simulink library "hcu_lib"  (Simulink 8.6)
settings: Solver=ode45  SolverMode=SingleTasking  StartTime=0.0  StopTime=10.0  RelTol=1e-3
PreLoadFcn:
  | if exist('tl_preloadfcn','file'), tl_preloadfcn(gcs,100); end
PostLoadFcn:
  | if exist('tl_postloadfcn','file'), tl_postloadfcn(gcs,100); end
undefined symbols (not defined in the file or in its folder): C_TICK_TIME_S, DEG2RAD, EPSILON, FALSE, RAD2DEG, TRUE
undefined symbols (not defined in the file): UNDEFINED_VALUE
libraries: hcu_lib x19, simulink x4
(part 2 of 3)

== system hcu_lib/P_Controller ==
  note: P Controller
  TargetValue : Inport
  FeedbackValue : Inport  Port=2
  FeedForward : Inport  Port=3
  Error_Gain : Inport  Port=4
  P_Gain : Inport  Port=5
  ControlHold : Inport  Port=6
  Constant14 : Constant  Value=single(0)
  Data Type Conversion : DataTypeConversion  OutDataTypeStr=single  SaturateOnIntegerOverflow=on  RndMeth=Zero
  Product2 : Product  InputSameDT=on  OutDataTypeStr=Inherit: Same as first input
  Product3 : Product  InputSameDT=on  OutDataTypeStr=Inherit: Same as first input
  Sum1 : Sum  Inputs=++|
  Sum2 : Sum  Inputs=+|-  SaturateOnIntegerOverflow=on  InputSameDT=on  OutDataTypeStr=Inherit: Same as first input
  Switch2 : Switch  Criteria=u2 ~= 0
  Switch4 : Switch  Criteria=u2 ~= 0
  Unit Delay1 : UnitDelay  SampleTime=-1
  Out : Outport  OutputWhenDisabled=reset  InitialOutput=[0]
  Control_Error : Outport  Port=2  OutputWhenDisabled=reset  InitialOutput=[0]
  P_term : Outport  Port=3  OutputWhenDisabled=reset  InitialOutput=[0]
  wires:
  FeedbackValue/1 -> Sum2/2
  TargetValue/1 -> Sum2/1
  Error_Gain/1 -> Product3/2
  P_Gain/1 -> Product2/1
  Product2/1 -> Sum1/2, P_term/1
  Product3/1 -> Product2/2
  Sum2/1 -> Data Type Conversion/1
  ControlHold/1 -> [HoldReq]
  [HoldReq] -> Switch2/2
  Switch2/1 -> Out/1, Unit Delay1/1
  Unit Delay1/1 -> Switch2/1
  Switch4/1 -> Product3/1
  Data Type Conversion/1 -> Control_Error/1, Switch4/3
  [HoldReq] -> Switch4/2
  Constant14/1 -> Switch4/1
  Sum1/1 -> Switch2/3
  FeedForward/1 -> Sum1/1

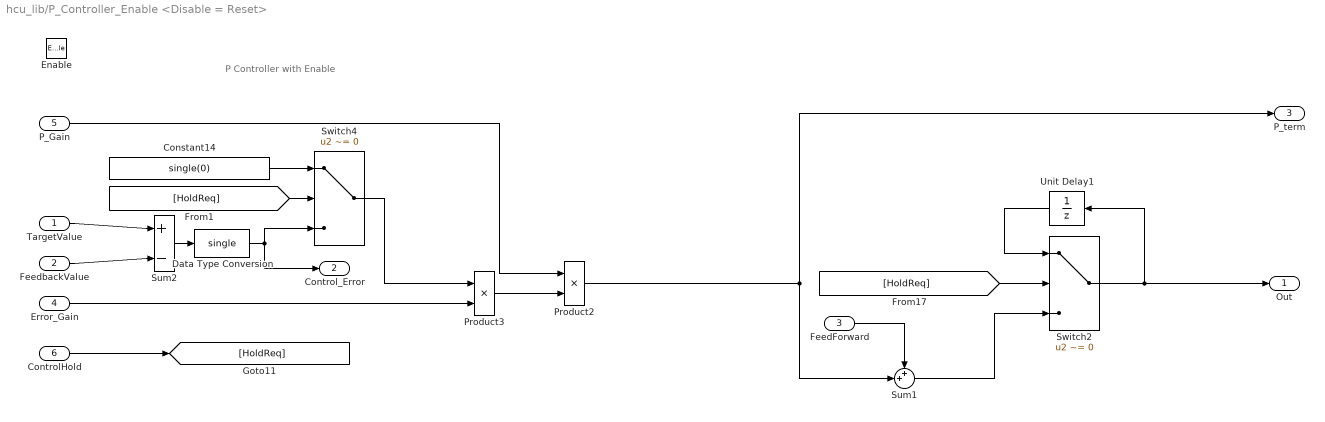
== system hcu_lib/P_Controller_Enable <Disable = Reset> ==
  note: P Controller with Enable
  TargetValue : Inport
  FeedbackValue : Inport  Port=2
  FeedForward : Inport  Port=3
  Error_Gain : Inport  Port=4
  P_Gain : Inport  Port=5
  ControlHold : Inport  Port=6
  Enable : EnablePort  StatesWhenEnabling=reset
  Constant14 : Constant  Value=single(0)
  Data Type Conversion : DataTypeConversion  OutDataTypeStr=single  SaturateOnIntegerOverflow=on  RndMeth=Zero
  Product2 : Product  InputSameDT=on  OutDataTypeStr=Inherit: Same as first input
  Product3 : Product  InputSameDT=on  OutDataTypeStr=Inherit: Same as first input
  Sum1 : Sum  Inputs=++|
  Sum2 : Sum  Inputs=+|-  SaturateOnIntegerOverflow=on  InputSameDT=on  OutDataTypeStr=Inherit: Same as first input
  Switch2 : Switch  Criteria=u2 ~= 0
  Switch4 : Switch  Criteria=u2 ~= 0
  Unit Delay1 : UnitDelay  SampleTime=-1
  Out : Outport  OutputWhenDisabled=reset  InitialOutput=[0]
  Control_Error : Outport  Port=2  OutputWhenDisabled=reset  InitialOutput=[0]
  P_term : Outport  Port=3  OutputWhenDisabled=reset  InitialOutput=[0]
  wires:
  FeedForward/1 -> Sum1/1
  Sum1/1 -> Switch2/3
  Constant14/1 -> Switch4/1
  [HoldReq] -> Switch4/2
  Data Type Conversion/1 -> Switch4/3, Control_Error/1
  Switch4/1 -> Product3/1
  Unit Delay1/1 -> Switch2/1
  Switch2/1 -> Unit Delay1/1, Out/1
  [HoldReq] -> Switch2/2
  ControlHold/1 -> [HoldReq]
  Sum2/1 -> Data Type Conversion/1
  Product3/1 -> Product2/2
  Product2/1 -> P_term/1, Sum1/2
  P_Gain/1 -> Product2/1
  Error_Gain/1 -> Product3/2
  TargetValue/1 -> Sum2/1
  FeedbackValue/1 -> Sum2/2

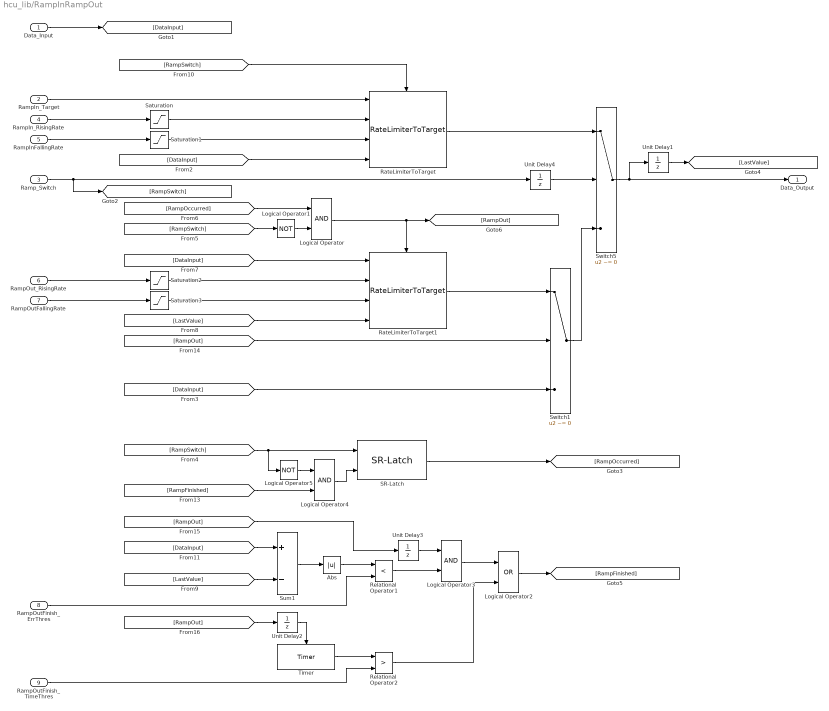
== system hcu_lib/RampInRampOut ==
  Data_Input : Inport
  RampIn_Target : Inport  Port=2
  Ramp_Switch : Inport  Port=3
  RampIn_RisingRate : Inport  Port=4
  RampInFallingRate : Inport  Port=5
  RampOut_RisingRate : Inport  Port=6
  RampOutFallingRate : Inport  Port=7
  RampOutFinish_ErrThres : Inport  Port=8
  RampOutFinish_TimeThres : Inport  Port=9
  Abs : Abs
  Logical Operator : Logic  AllPortsSameDT=off  OutDataTypeStr=boolean
  Logical Operator1 : Logic  Operator=NOT  AllPortsSameDT=off  OutDataTypeStr=boolean
  Logical Operator2 : Logic  Operator=OR  AllPortsSameDT=off  OutDataTypeStr=boolean
  Logical Operator3 : Logic  AllPortsSameDT=off  OutDataTypeStr=boolean
  Logical Operator4 : Logic  AllPortsSameDT=off  OutDataTypeStr=boolean
  Logical Operator5 : Logic  Operator=NOT  AllPortsSameDT=off  OutDataTypeStr=boolean
  RateLimiterToTarget : hcu_lib/RateLimiterToTarget  SystemSampleTime=-1
  RateLimiterToTarget1 : hcu_lib/RateLimiterToTarget  SystemSampleTime=-1
  Relational Operator1 : RelationalOperator  Operator=<  OutDataTypeStr=boolean
  Relational Operator2 : RelationalOperator  Operator=>  OutDataTypeStr=boolean
  SR-Latch : hcu_lib/SR-Latch  SystemSampleTime=-1
  Saturation : Saturate  UpperLimit=inf  LowerLimit=0
  Saturation1 : Saturate  UpperLimit=0  LowerLimit=-inf
  Saturation2 : Saturate  UpperLimit=inf  LowerLimit=0
  Saturation3 : Saturate  UpperLimit=0  LowerLimit=-inf
  Sum1 : Sum  Inputs=+-
  Switch1 : Switch  Criteria=u2 ~= 0
  Switch5 : Switch  Criteria=u2 ~= 0
  Timer : hcu_lib/Timer  SystemSampleTime=-1
  Unit Delay{1..4} (4 alike) : UnitDelay  SampleTime=-1
  Data_Output : Outport  InitialOutput=[0]
  wires:
  Data_Input/1 -> [DataInput]
  RateLimiterToTarget/1 -> Switch5/1
  [RampSwitch] -> RateLimiterToTarget/Enable
  RampIn_Target/1 -> RateLimiterToTarget/1
  RampIn_RisingRate/1 -> Saturation/1
  RampInFallingRate/1 -> Saturation1/1
  [DataInput] -> RateLimiterToTarget/4
  [DataInput] -> Switch1/3
  Switch5/1 -> Unit Delay1/1, Data_Output/1
  [RampSwitch] -> SR-Latch/1, Logical Operator5/1
  SR-Latch/1 -> [RampOccurred]
  Switch1/1 -> Switch5/3
  [RampSwitch] -> Logical Operator1/1
  [RampOccurred] -> Logical Operator/1
  Logical Operator1/1 -> Logical Operator/2
  [DataInput] -> RateLimiterToTarget1/1
  RampOut_RisingRate/1 -> Saturation2/1
  RampOutFallingRate/1 -> Saturation3/1
  [LastValue] -> RateLimiterToTarget1/4
  Unit Delay1/1 -> [LastValue]
  [DataInput] -> Sum1/1
  [LastValue] -> Sum1/2
  Sum1/1 -> Abs/1
  Abs/1 -> Relational Operator1/1
  RampOutFinish_ErrThres/1 -> Relational Operator1/2
  [RampOut] -> Unit Delay2/1
  Timer/1 -> Relational Operator2/1
  RampOutFinish_TimeThres/1 -> Relational Operator2/2
  Relational Operator1/1 -> Logical Operator3/2
  Relational Operator2/1 -> Logical Operator2/2
  Logical Operator2/1 -> [RampFinished]
  [RampFinished] -> Logical Operator4/2
  Unit Delay2/1 -> Timer/Enable
  Logical Operator3/1 -> Logical Operator2/1
  Logical Operator5/1 -> Logical Operator4/1
  Logical Operator4/1 -> SR-Latch/2
  Logical Operator/1 -> RateLimiterToTarget1/Enable, [RampOut]
  Ramp_Switch/1 -> Unit Delay4/1, [RampSwitch]
  RateLimiterToTarget1/1 -> Switch1/1
  Unit Delay4/1 -> Switch5/2
  [RampOut] -> Switch1/2
  Unit Delay3/1 -> Logical Operator3/1
  [RampOut] -> Unit Delay3/1
  Saturation/1 -> RateLimiterToTarget/2
  Saturation1/1 -> RateLimiterToTarget/3
  Saturation3/1 -> RateLimiterToTarget1/3
  Saturation2/1 -> RateLimiterToTarget1/2

== system hcu_lib/RateLimit ==
  input_raw : Inport
  steptime : Inport  Port=2
  ratelimt_inc : Inport  Port=3
  ratelimt_dec : Inport  Port=4
  MinMax : MinMax  Inputs=2
  MinMax1 : MinMax  Function=max  Inputs=2
  MinMax2 : MinMax  Function=max  Inputs=2
  MinMax3 : MinMax  Inputs=2
  Product : Product  RndMeth=Zero
  Product1 : Product  RndMeth=Zero
  Sum5 : Sum  Inputs=+-
  Sum6 : Sum
  UnitDelay1 : UnitDelay  SampleTime=-1
  step_time6 : Constant  Value=0  OutDataTypeStr=single
  output : Outport
  wires:
  ratelimt_dec/1 -> Product1/2
  steptime/1 -> Product1/1, Product/2
  Sum5/1 -> MinMax1/1
  [Dec] -> MinMax1/2
  [Inc] -> MinMax/1
  MinMax1/1 -> MinMax/2
  MinMax/1 -> Sum6/1
  input_raw/1 -> Sum5/1
  Sum6/1 -> output/1, UnitDelay1/1
  UnitDelay1/1 -> Sum5/2, Sum6/2
  Product/1 -> MinMax2/1
  Product1/1 -> MinMax3/2
  step_time6/1 -> MinMax2/2, MinMax3/1
  MinMax2/1 -> [Inc]
  MinMax3/1 -> [Dec]
  ratelimt_inc/1 -> Product/1

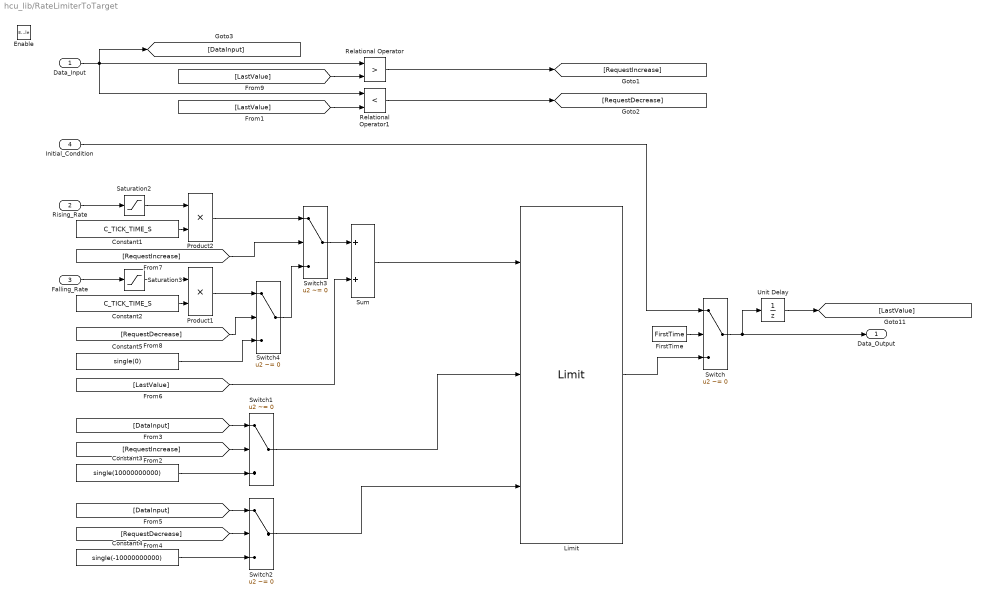
== system hcu_lib/RateLimiterToTarget ==
  Data_Input : Inport
  Rising_Rate : Inport  Port=2
  Falling_Rate : Inport  Port=3
  Initial_Condition : Inport  Port=4
  Enable : EnablePort  StatesWhenEnabling=reset
  Constant1 : Constant  Value=C_TICK_TIME_S
  Constant2 : Constant  Value=C_TICK_TIME_S
  Constant3 : Constant  Value=single(10000000000)
  Constant4 : Constant  Value=single(-10000000000)
  Constant5 : Constant  Value=single(0)
  FirstTime : hcu_lib/FirstTime
  Limit : hcu_lib/Limit  SystemSampleTime=-1
  Product1 : Product  Inputs=**  RndMeth=Zero
  Product2 : Product  Inputs=**  RndMeth=Zero
  Relational Operator : RelationalOperator  Operator=>  OutDataTypeStr=boolean
  Relational Operator1 : RelationalOperator  Operator=<  OutDataTypeStr=boolean
  Saturation2 : Saturate  UpperLimit=inf  LowerLimit=0
  Saturation3 : Saturate  UpperLimit=0  LowerLimit=-inf
  Sum : Sum
  Switch{,1..4} (5 alike) : Switch  Criteria=u2 ~= 0
  Unit Delay : UnitDelay  SampleTime=-1
  Data_Output : Outport  InitialOutput=[0]
  wires:
  Limit/1 -> Switch/3
  Saturation3/1 -> Product1/1
  Saturation2/1 -> Product2/1
  Constant5/1 -> Switch4/3
  Product1/1 -> Switch4/1
  Switch4/1 -> Switch3/3
  [RequestDecrease] -> Switch4/2
  Switch3/1 -> Sum/1
  Product2/1 -> Switch3/1
  [LastValue] -> Sum/2
  [RequestIncrease] -> Switch3/2
  Switch2/1 -> Limit/3
  Switch1/1 -> Limit/2
  [DataInput] -> Switch2/1
  Constant4/1 -> Switch2/3
  [RequestDecrease] -> Switch2/2
  Constant3/1 -> Switch1/3
  [DataInput] -> Switch1/1
  [RequestIncrease] -> Switch1/2
  Switch/1 -> Data_Output/1, Unit Delay/1
  Relational Operator1/1 -> [RequestDecrease]
  [LastValue] -> Relational Operator1/2
  Data_Input/1 -> Relational Operator1/1, Relational Operator/1, [DataInput]
  Relational Operator/1 -> [RequestIncrease]
  [LastValue] -> Relational Operator/2
  Unit Delay/1 -> [LastValue]
  Falling_Rate/1 -> Saturation3/1
  Constant2/1 -> Product1/2
  Rising_Rate/1 -> Saturation2/1
  Sum/1 -> Limit/1
  Initial_Condition/1 -> Switch/1
  FirstTime/1 -> Switch/2
  Constant1/1 -> Product2/2

== system hcu_lib/ReqId ==

== system hcu_lib/SIN ==
  u_rad : Inport
  Constant : Constant  Value=single(2*pi)
  Gain : Gain  Gain=2*pi
  Product : Product  Inputs=*/
  Rounding Function : Rounding
  SIN_Function : Lookup_n-D  NumberOfTableDimensions=1  BreakpointsForDimension1="[0\t5\t10\t15\t30\t45\t60\t75\t80\t85\t90\t95\t100\t105\t120\t135\t150\t165\t170\t175\t180\t185\t190\t195\t210\t225\t240\t255\t260\t265\t270\t275\t280\t285\t300\t315\t330\t345\t350\t355\t360]"  Table="[0\t0.087155743\t0.173648178\t0.258819045\t0.5\t0.707106781\t0.866025404\t0.965925826\t0.984807753\t0.996194698\t1\t0.996194698\t0.984807753\t0.965925826\t0.866025404\t0.707106781\t0.5\t0.258819045\t0.173648178\t0.087155743\t0\t-0.087155743\t-0.173648178\t-0.258819045\t-0.5\t-0.707106781\t-0.866025404\t-0.965925826\t-0.984807753\t-0.996194698\t-1\t-0.996194698\t-0.984807753\t-0.965925826\t-0.866025404\t-0.707106781\t-0.5\t-0.258819045\t-0.173648178\t-0.087155743\t0]"  ExtrapMethod=Clip  UseLastTableValue=on  InternalRulePriority=Speed  RndMeth=Simplest  InputSameDT=on
  Saturation : Saturate  UpperLimit=360  LowerLimit=0
  Subtract : Sum  Inputs=+-
  km2miles1 : Subsystem  mask(Conversion){}
      mask help: Convert rads to degs.
      mask Display: disp('rad \rightarrow deg', 'texmode', 'on')
  y : Outport
  wires:
  SIN_Function/1 -> y/1
  Saturation/1 -> SIN_Function/1
  km2miles1/1(y) -> Saturation/1
  u_rad/1 -> Product/1, Subtract/1
  Constant/1 -> Product/2
  Product/1 -> Rounding Function/1
  Rounding Function/1 -> Gain/1
  Gain/1 -> Subtract/2
  Subtract/1 -> km2miles1/1(u)

== system hcu_lib/SR-Latch ==
  set : Inport
  reset : Inport  Port=2
  Logical Operator : Logic  AllPortsSameDT=off  OutDataTypeStr=boolean
  Logical Operator1 : Logic  Operator=NOT  AllPortsSameDT=off  OutDataTypeStr=boolean
  Switch1 : Switch  Criteria=u2 ~= 0  Threshold=0.5
      settings: AttributesFormatString=<Criteria=%<Criteria>>
  Switch2 : Switch  Criteria=u2 ~= 0  Threshold=0.5
      settings: AttributesFormatString=<Criteria=%<Criteria>>
  Unit Delay : UnitDelay  SampleTime=-1
  latched : Outport
  wires:
  Logical Operator1/1 -> Switch2/1, Logical Operator/2
  Logical Operator/1 -> Switch1/2
  Switch2/1 -> Switch1/3
  Unit Delay/1 -> Switch2/3
  reset/1 -> Logical Operator1/1, Switch2/2
  set/1 -> Logical Operator/1, Switch1/1
  Switch1/1 -> latched/1, Unit Delay/1

== system hcu_lib/Signal_Conversion_Blocks ==
  Raw32 : Subsystem  TreatAsAtomicUnit=on  RTWFcnName=raw32_lib  RTWFileName=HCU_LIB  mask(RawDataConversion){}
      mask help: Raw data conversion.
      settings: RTWFcnNameOpts=User specified  RTWFileNameOpts=User specified
  conv_counts_to_eng_units : Subsystem  TreatAsAtomicUnit=on  RTWFcnName=convcountstoengunits_lib  RTWFileName=HCU_LIB  mask(Signal Conversion){}
      mask help: Converts counts to engineering units.
      settings: RTWFcnNameOpts=User specified  RTWFileNameOpts=User specified
  conv_eng_units_to_counts : Subsystem  TreatAsAtomicUnit=on  RTWFcnName=convengunitstocounts_lib  RTWFileName=HCU_LIB  mask(Signal Conversion){}
      mask help: Converts engineering units to counts.
      settings: RTWFcnNameOpts=User specified  RTWFileNameOpts=User specified
  convert_in : Subsystem  TreatAsAtomicUnit=on  RTWFcnName=convertin_lib  RTWFileName=HCU_LIB  mask(ConvertIn){gain=UNDEFINED_VALUE, offset=UNDEFINED_VALUE}
      mask help:
      | Conversion Formula
      |
      | The conversion formula is
      |
      | raw_value = (physical_value - Offset) / Factor
      |
      | where physical_value is the value of the signal after it is saturated using the specified Min and Max values. raw_value is the packed signal value.
      settings: AttributesFormatString=gain : %<gain> / offset : %<offset>  RTWFcnNameOpts=User specified  RTWFileNameOpts=User specified
  convert_out : Subsystem  TreatAsAtomicUnit=on  RTWFcnName=convertout_lib  RTWFileName=HCU_LIB  mask(ConvertOut){gain=UNDEFINED_VALUE, offset=UNDEFINED_VALUE}
      mask help:
      | Conversion Formula
      |
      | The conversion formula is
      |
      | raw_value = (physical_value - Offset) / Factor
      |
      | where physical_value is the value of the signal after it is saturated using the specified Min and Max values. raw_value is the packed signal value.
      settings: RTWFcnNameOpts=User specified  RTWFileNameOpts=User specified

== system hcu_lib/Signal_over ==
  u : Inport
  Data Type Conversion : DataTypeConversion
  If : If  IfExpression=u1 ~= 0
  Merge : Merge
  NewValue : Subsystem
  OldValue : Subsystem
  override_cal : Constant  Value=cal  OutDataTypeStr=Inherit: Inherit via back propagation
  override_enable : Constant  Value=0  OutDataTypeStr=boolean
  y : Outport
  wires:
  override_cal/1 -> NewValue/1(In1)
  If/2 -> OldValue/Action
  If/1 -> NewValue/Action
  override_enable/1 -> If/1
  OldValue/1(Out1) -> Merge/2
  NewValue/1(Out1) -> Merge/1
  Merge/1 -> Data Type Conversion/1  "y"
  u/1 -> OldValue/1(In1)  "u"
  Data Type Conversion/1 -> y/1

== system hcu_lib/TAN ==
  u_rad : Inport
  COS : Subsystem  TreatAsAtomicUnit=on  mask(Cosine function){}
      mask help:
      | Calculate Cosine of the Input Signal.
      | The unit of input signal is rad.
      settings: RTWFcnNameOpts=Use subsystem name  RTWFileNameOpts=Use subsystem name
      mask Display:
      | disp('       COS(X)' , 'texmode', 'on');
      | port_label('output',1,'Y');
      | port_label('input',1,'X_rad')
  Product : Product  Inputs=*/
  SIN : Subsystem  TreatAsAtomicUnit=on  mask(Sine function){}
      mask help:
      | Calculate Sine of the Input Signal.
      | The unit of input signal is rad.
      settings: RTWFcnNameOpts=Use subsystem name  RTWFileNameOpts=Use subsystem name
      mask Display:
      | disp('      SIN(X)' , 'texmode', 'on');
      | port_label('output',1,'Y');
      | port_label('input',1,'X_rad')
  y : Outport
  wires:
  COS/1(y) -> Product/2
  u_rad/1 -> COS/1(u_rad), SIN/1(u_rad)
  SIN/1(y) -> Product/1
  Product/1 -> y/1

== system hcu_lib/Timer ==
  Enable : EnablePort  StatesWhenEnabling=reset  ZeroCross=off
  Constant : Constant  Value=C_TICK_TIME_S
  Sum : Sum  Inputs=|++  SaturateOnIntegerOverflow=on  InputSameDT=on
  Unit Delay : UnitDelay  SampleTime=-1
  Timer (sec) : Outport  OutputWhenDisabled=reset  InitialOutput=0
  wires:
  Unit Delay/1 -> Timer (sec)/1, Sum/2
  Sum/1 -> Unit Delay/1
  Constant/1 -> Sum/1

== system hcu_lib/deg2rad ==
  u : Inport
  Gain : Gain  Gain=pi/180
  y : Outport
  wires:
  Gain/1 -> y/1  "y"
  u/1 -> Gain/1  "u"

== system hcu_lib/divide ==
  dividend : Inport
  divisor : Inport  Port=2
  default_value : Inport  Port=3
  Divide : Product  Inputs=*/
  Interval Test : simulink/Logic and Bit Operations/Interval Test  IntervalClosedRight=on  uplimit=0.00001  IntervalClosedLeft=on  lowlimit=-0.00001  OutDataTypeStr=boolean
  Logical Operator : Logic  Operator=NOT  Inputs=1  AllPortsSameDT=off  OutDataTypeStr=boolean
  Switch : Switch  Criteria=u2 ~= 0  Threshold=0.5
  quotient : Outport
  wires:
  Logical Operator/1 -> Switch/2
  default_value/1 -> Switch/3  "default_value"
  Interval Test/1 -> Logical Operator/1
  Switch/1 -> quotient/1
  Divide/1 -> Switch/1
  divisor/1 -> Interval Test/1, Divide/2  "divisor"
  dividend/1 -> Divide/1  "dividend"

== system hcu_lib/fault_filter_latch ==
  i_fault : Inport
  sat : Inport  Port=2
  inc : Inport  Port=3
  dec : Inport  Port=4
  Add : Sum
  Constant : Constant  Value=0  OutDataTypeStr=Inherit: Inherit via back propagation
  Data Type Conversion : DataTypeConversion  OutDataTypeStr=int16
  Gain : Gain  Gain=-1
  MinMax : MinMax  Function=max  Inputs=2
  MinMax1 : MinMax  Inputs=2
  Relational Operator : RelationalOperator  OutDataTypeStr=boolean
  Switch : Switch
  Switch1 : Switch
  Unit Delay : UnitDelay  SampleTime=-1
  Unit Delay1 : UnitDelay  SampleTime=-1
  fault_flg : Outport
  ff_count : Outport  Port=2
  wires:
  inc/1 -> Switch/1  "inc"
  dec/1 -> Gain/1  "dec"
  i_fault/1 -> Switch/2  "i_fault"
  Switch/1 -> Add/1
  Unit Delay/1 -> Add/2
  Gain/1 -> Switch/3
  Add/1 -> Data Type Conversion/1
  Constant/1 -> MinMax/2
  MinMax/1 -> MinMax1/1
  MinMax1/1 -> ff_count/1, Unit Delay/1, Relational Operator/1
  sat/1 -> MinMax1/2, Relational Operator/2  "sat"
  Relational Operator/1 -> Switch1/2, Switch1/1
  Switch1/1 -> fault_flg/1, Unit Delay1/1
  Unit Delay1/1 -> Switch1/3
  Data Type Conversion/1 -> MinMax/1

== system hcu_lib/fault_filter_reset ==
  i_fault : Inport
  sat : Inport  Port=2
  inc : Inport  Port=3
  dec : Inport  Port=4
  Add : Sum
  Add1 : Sum  Inputs=+-
  Constant : Constant  Value=0  OutDataTypeStr=uint8
  Data Type Conversion : DataTypeConversion  OutDataTypeStr=int16
  MinMax : MinMax  Function=max  Inputs=2
  MinMax1 : MinMax  Inputs=2
  Relational Operator : RelationalOperator  OutDataTypeStr=boolean
  Switch : Switch  Criteria=u2 ~= 0
  Unit Delay : UnitDelay  SampleTime=-1
  fault_flg : Outport
  ff_count : Outport  Port=2
  wires:
  inc/1 -> Add/2  "inc"
  dec/1 -> Add1/2  "dec"
  i_fault/1 -> Switch/2  "i_fault"
  Unit Delay/1 -> Add/1, Add1/1
  Constant/1 -> MinMax/2
  MinMax/1 -> MinMax1/1
  MinMax1/1 -> ff_count/1, Unit Delay/1, Relational Operator/1
  sat/1 -> MinMax1/2, Relational Operator/2  "sat"
  Relational Operator/1 -> fault_flg/1
  Add/1 -> Switch/1
  Add1/1 -> Switch/3
  Switch/1 -> Data Type Conversion/1
  Data Type Conversion/1 -> MinMax/1

== system hcu_lib/km2miles ==
  u : Inport
  Gain : Gain  Gain=1/1.6093
  y : Outport
  wires:
  Gain/1 -> y/1  "y"
  u/1 -> Gain/1  "u"

== system hcu_lib/kph2mps ==
  u : Inport
  Gain : Gain  Gain=1000/3600
  y : Outport
  wires:
  Gain/1 -> y/1  "y"
  u/1 -> Gain/1  "u"

== system hcu_lib/kxx2xx ==
  u : Inport
  Gain : Gain  Gain=1000
  y : Outport
  wires:
  u/1 -> Gain/1  "u"
  Gain/1 -> y/1  "y"

== system hcu_lib/latching fault filter reinit ==
  i_fault : Inport
  sat : Inport  Port=2
  inc : Inport  Port=3
  dec : Inport  Port=4
  reinit : Inport  Port=5
  lff_ctl : Stateflow chart  TreatAsAtomicUnit=on
  fault_flg : Outport
  ff_count : Outport  Port=2
  wires:
  dec/1 -> lff_ctl/3(dec)  "dec"
  i_fault/1 -> lff_ctl/4(i_fault)  "i_fault"
  lff_ctl/1(fault_flg) -> fault_flg/1  "fault_flg"
  inc/1 -> lff_ctl/2(inc)  "inc"
  sat/1 -> lff_ctl/1(sat)  "sat"
  lff_ctl/2(ff_count) -> ff_count/1  "ff_count"
  reinit/1 -> lff_ctl/5(reinit)  "reinit"

== system hcu_lib/latching_fault_filter ==
  i_fault : Inport
  sat : Inport  Port=2
  inc : Inport  Port=3
  dec : Inport  Port=4
  lff_ctl : Stateflow chart  TreatAsAtomicUnit=on
  fault_flg : Outport
  ff_count : Outport  Port=2
  wires:
  dec/1 -> lff_ctl/3(dec)  "dec"
  i_fault/1 -> lff_ctl/4(i_fault)  "i_fault"
  lff_ctl/1(fault_flg) -> fault_flg/1  "fault_flg"
  inc/1 -> lff_ctl/2(inc)  "inc"
  sat/1 -> lff_ctl/1(sat)  "sat"
  lff_ctl/2(ff_count) -> ff_count/1  "ff_count"

== system hcu_lib/litres2gallons ==
  u : Inport
  Constant : Constant  Value=UK  OutDataTypeStr=boolean
  Switch : Switch  Threshold=0.5  ZeroCross=off
  UK : Gain  Gain=0.2199692483
  US : Gain  Gain=0.2641720524
  y : Outport
  wires:
  UK/1 -> Switch/1
  US/1 -> Switch/3
  u/1 -> UK/1, US/1  "u"
  Switch/1 -> y/1  "y"
  Constant/1 -> Switch/2

== system hcu_lib/miles2km ==
  u : Inport
  Gain : Gain  Gain=1.6093
  y : Outport
  wires:
  u/1 -> Gain/1  "u"
  Gain/1 -> y/1  "y"

== system hcu_lib/miles2km1 ==
  u : Inport
  Gain : Gain  Gain=DEG2RAD
  y : Outport
  wires:
  Gain/1 -> y/1  "y"
  u/1 -> Gain/1  "u"

== system hcu_lib/mps22G ==
  u : Inport
  Gain : Gain  Gain=1/9.81
  y : Outport
  wires:
  u/1 -> Gain/1  "u"
  Gain/1 -> y/1  "y"

== system hcu_lib/mps2kph ==
  u : Inport
  Gain : Gain  Gain=3600/1000
  y : Outport
  wires:
  u/1 -> Gain/1  "u"
  Gain/1 -> y/1  "y"

== system hcu_lib/override signal ==
  note: When either service_ovrdflg or cal_ovrdflg is true, signal_valid_flg is set as TRUE
  note: ONLY ONE ovrdflg (Service_ovrdflg and Cal_ovrdflg) can be valid
      | Set the priority of Service_ovrdflg higher than Cal_ovrdflg
      | In this way, the Cal_ovrd can be automatically disabled in production
  signal_valid_flg_raw : Inport
  signal_raw : Inport  Port=2
  service_ovrdflg : Inport  Port=3
  service_ovrdval : Inport  Port=4
  cal_ovrdflg : Inport  Port=5
  cal_ovrdval : Inport  Port=6
  Data Type Duplicate : DataTypeDuplicate  NumInputPorts=5
  Logical Operator : Logic  Operator=OR  AllPortsSameDT=off  OutDataTypeStr=boolean
  Switch : Switch  Criteria=u2 ~= 0  Threshold=0.5
  Switch1 : Switch  Criteria=u2 ~= 0  Threshold=0.5
  Switch2 : Switch  Criteria=u2 ~= 0  Threshold=0.5
  True : Constant  Value=TRUE  OutDataTypeStr=boolean
  signal : Outport
  signal_valid_flg : Outport  Port=2
  wires:
  signal_valid_flg_raw/1 -> Switch2/3  "signal_valid_flg_raw"
  Switch2/1 -> signal_valid_flg/1  "signal_valid_flg"
  True/1 -> Switch2/1
  Logical Operator/1 -> Switch2/2
  Switch1/1 -> Switch/3, Data Type Duplicate/4
  signal_raw/1 -> Switch1/3, Data Type Duplicate/1  "signal_raw"
  cal_ovrdval/1 -> Switch1/1, Data Type Duplicate/2  "cal_ovrdval"
  service_ovrdval/1 -> Switch/1, Data Type Duplicate/3  "service_ovrdval"
  cal_ovrdflg/1 -> Switch1/2, [cal_ovrdflg]  "cal_ovrdflg"
  service_ovrdflg/1 -> Switch/2, [service_ovrdflg]  "service_ovrdflg"
  Switch/1 -> signal/1, Data Type Duplicate/5  "signal"
  [service_ovrdflg] -> Logical Operator/1
  [cal_ovrdflg] -> Logical Operator/2

== system hcu_lib/rad2deg ==
  u : Inport
  Gain : Gain  Gain=180/pi
  y : Outport
  wires:
  u/1 -> Gain/1  "u"
  Gain/1 -> y/1  "y"

== system hcu_lib/radps2rpm ==
  u : Inport
  Gain : Gain  Gain=60/2/pi
  y : Outport
  wires:
  u/1 -> Gain/1  "u"
  Gain/1 -> y/1  "y"

== system hcu_lib/rolling average ==
  note: Using the first two terms of the series expansion:
      |
      |                     x                     x2
      |                                e   =  1  +  x  +  --  + ......
      |                                           2!
      |
      |       Simplifying, the exponential "f" becomes:
      |
      |                  - (FK_TMR/TC)              1
      |           f  =  1  -  e                    =  1  -  -------------  =  . . .
      |                                                    (FK_TMR/TC)
      |                           e
      |
      |                              1                      1
      |          f  =  1  -  ---------------------------------  =    ------------------- .
      |                                  1 + (FK_TMR / TC)       1 + (TC / FK_TMR)
  note: - (FK_TMR/TC)
      |                                    f  =  1  -  e
      |
      |       Where "f" is called the filter constant in the difference equation:
      |
      |                    new_average = f * new_value + (1 - f) * old_average
  note: new_average = [ (sample_interval)/(sample_interval + time_constant) ] * (new_value - old_ave) + old_ave
  new_value : Inport
  old_ave : Inport  Port=2
  delta_t : Inport  Port=3
  tc : Inport  Port=4
  IC : UnitDelay  Tag=struct('comment',struct('text','','placement',1),'logdata',struct('maxnumvals',inf,'plotchannels',[],'stepsize',0,'downsampling',1,'loggingmode',3,'channels',1),'output',struct('width',1,'name','$S_$B','unit','','type','Int16','offset',0,'max',NaN,'min',NaN,'freeze',1,'lsb',1,'arb',0,'class','default','address','','description','','autoscalingmode',1,'lowerheadroom',1,'upperheadroom',1,'headroomunit','bit','checkmin',0,'checkmax',0,'show',0,'initial','2'),'state',0,'dt','-1','date',731455.586925799)  InitialCondition=1  SampleTime=-1
  Product_tmp1 : Product  Tag=struct('comment',struct('text','','placement',1),'logdata',struct('maxnumvals',inf,'plotchannels',[],'stepsize',0,'downsampling',1,'loggingmode',3,'channels',1),'output',struct('width',1,'name','$S_$B','unit','','type','Int32Bin15','offset',0,'max',65535,'min',-65536,'freeze',1,'lsb',2^-15,'arb',0,'class','default','address','','description','','autoscalingmode',1,'lowerheadroom',1,'upperheadroom',1,'headroomunit','bit','checkmin',0,'checkmax',0,'show',0),'inputs','**','exceptionhandling',1,'date',731455.58640515)  Inputs=**  RndMeth=Zero  InputSameDT=on  OutDataTypeStr=Inherit: Same as first input
  Sum : Sum  Tag=struct('comment',struct('text','','placement',1),'logdata',struct('maxnumvals',inf,'plotchannels',[],'stepsize',0,'downsampling',1,'loggingmode',3,'channels',1),'output',struct('width',1,'name','$S_$B','unit','','type','Int32Bin15','offset',0,'max',65535,'min',-65536,'freeze',1,'lsb',2^-15,'arb',0,'class','default','address','','description','','autoscalingmode',1,'lowerheadroom',1,'upperheadroom',1,'headroomunit','bit','checkmin',0,'checkmax',0,'show',0),'inputs','-+','date',731455.586330463)  Inputs=-+  InputSameDT=on  OutDataTypeStr=Inherit: Same as first input
  Sum1 : Sum  Tag=struct('comment',struct('text','','placement',1),'logdata',struct('maxnumvals',inf,'plotchannels',[],'stepsize',0,'downsampling',1,'loggingmode',3,'channels',1),'output',struct('width',1,'name','$S_$B','unit','','type','Int32Bin15','offset',0,'max',65535,'min',-65536,'freeze',1,'lsb',2^-15,'arb',0,'class','default','address','','description','','autoscalingmode',1,'lowerheadroom',1,'upperheadroom',1,'headroomunit','bit','checkmin',0,'checkmax',0,'show',0),'inputs','++','date',731455.58628235)  InputSameDT=on  OutDataTypeStr=Inherit: Same as first input
  Sum2 : Sum  Tag=struct('comment',struct('text','','placement',1),'logdata',struct('maxnumvals',inf,'plotchannels',[],'stepsize',0,'downsampling',1,'loggingmode',3,'channels',1),'output',struct('width',1,'name','$S_$B','unit','','type','Int32Bin15','offset',0,'max',65535,'min',-65536,'freeze',1,'lsb',2^-15,'arb',0,'class','default','address','','description','','autoscalingmode',1,'lowerheadroom',1,'upperheadroom',1,'headroomunit','bit','checkmin',0,'checkmax',0,'show',0),'inputs','++','date',731455.586506424)  InputSameDT=on  OutDataTypeStr=Inherit: Same as first input
  Switch1 : Switch  Tag=struct('comment',struct('text','','placement',1),'logdata',struct('maxnumvals',inf,'plotchannels',[],'stepsize',0,'downsampling',1,'loggingmode',3,'channels',1),'output',struct('width',1,'name','$S_$B','unit','','type','Int32Bin15','offset',0,'max',65535,'min',-65536,'freeze',1,'lsb',2^-15,'arb',0,'class','default','address','','description','','autoscalingmode',1,'lowerheadroom',1,'upperheadroom',1,'headroomunit','bit','checkmin',0,'checkmax',0,'show',0),'threshold',struct('width',1,'name','$S_$B_threshold','unit','','type','Int16','offset',0,'max',NaN,'min',NaN,'freeze',1,'lsb',1,'arb',0,'class','default','address','','description','','value','1','scalar',0),'date',731455.58657044)  Threshold=0.5  InputSameDT=on
  divide : hcu_lib/divide
  zero : Constant  Tag=struct('comment',struct('text','','placement',1),'output',struct('width',1,'name','$S_$B','unit','','type','Int16','offset',0,'max',NaN,'min',NaN,'freeze',1,'lsb',1,'arb',0,'class','default','address','','description','','value','0','tolerance',1,'show',0),'date',731455.58675544)  Value=0  OutDataTypeStr=Inherit: Inherit via back propagation
  zero1 : Constant  Tag=struct('comment',struct('text','','placement',1),'output',struct('width',1,'name','$S_$B','unit','','type','Int16','offset',0,'max',NaN,'min',NaN,'freeze',1,'lsb',1,'arb',0,'class','default','address','','description','','value','0','tolerance',1,'show',0),'date',731455.58675544)  Value=0  OutDataTypeStr=Inherit: Inherit via back propagation
  new_ave : Outport
  wires:
  old_ave/1 -> Sum/1, Sum2/1  "old_ave"
  new_value/1 -> [new_value], Sum/2  "new_value"
  delta_t/1 -> Sum1/1, Product_tmp1/2  "delta_t"
  tc/1 -> Sum1/2
  divide/1 -> Sum2/2
  Sum/1 -> Product_tmp1/1
  Sum1/1 -> divide/2
  zero/1 -> IC/1
  IC/1 -> Switch1/2
  Sum2/1 -> Switch1/3  "new_ave"
  Switch1/1 -> new_ave/1  "new_ave"
  [new_value] -> Switch1/1
  Product_tmp1/1 -> divide/1
  zero1/1 -> divide/3

== system hcu_lib/rpm2radps ==
  u : Inport
  Gain : Gain  Gain=2*pi/60
  y : Outport
  wires:
  Gain/1 -> y/1  "y"
  u/1 -> Gain/1  "u"

== system hcu_lib/saturate_dynamic ==
  up : Inport
  u : Inport  Port=2
  lo : Inport  Port=3
  LowerRelop1 : RelationalOperator  DisableCoverage=on  Operator=>  OutDataTypeStr=boolean
  Switch : Switch  Criteria=u2 ~= 0  Threshold=0.5  OutDataTypeStr=Inherit: Inherit via back propagation  ZeroCross=off
  Switch2 : Switch  Criteria=u2 ~= 0  Threshold=0.5  OutDataTypeStr=Inherit: Inherit via back propagation  ZeroCross=off
  UpperRelop : RelationalOperator  DisableCoverage=on  Operator=<  OutDataTypeStr=boolean
  y : Outport
  wires:
  [up] -> Switch2/1  "up"
  [up] -> LowerRelop1/2  "up"
  up/1 -> [up]  "up"
  [lo] -> Switch/1  "lo"
  lo/1 -> [lo]  "lo"
  [u] -> UpperRelop/1  "u"
  [u] -> LowerRelop1/1  "u"
  u/1 -> [u]  "u"
  [u] -> Switch/3  "u"
  [lo] -> UpperRelop/2  "lo"
  Switch/1 -> Switch2/3
  Switch2/1 -> y/1
  LowerRelop1/1 -> Switch2/2
  UpperRelop/1 -> Switch/2

== system hcu_lib/sig_valid_check ==
  new_signal : Inport
  new_signal_valid_flg : Inport  Port=2
  invalid_override : Inport  Port=3
  valid_override : Inport  Port=4
  def_value : Inport  Port=5
  sat : Inport  Port=6
  inc : Inport  Port=7
  dec : Inport  Port=8
  Logical Operator : Logic  Tag=struct('inputs','2','comment',struct('text','','placement',1),'logdata',struct('maxnumvals',inf,'plotchannels',[],'stepsize',0,'downsampling',1,'loggingmode',3,'channels',1),'operator','OR','output',struct('class','default','type','Bool8','description','','address','','unit','','name','$S_$B'),'date',731430.467498704)
  Logical Operator1 : Logic  Tag=struct('inputs','1','comment',struct('text','','placement',1),'logdata',struct('maxnumvals',inf,'plotchannels',[],'stepsize',0,'downsampling',1,'loggingmode',3,'channels',1),'operator','NOT','output',struct('class','default','type','Bool8','description','','address','','unit','','name','$S_$B'),'date',731430.46749816)  Operator=NOT  Inputs=1
  Logical Operator2 : Logic  Tag=struct('inputs','1','comment',struct('text','','placement',1),'logdata',struct('maxnumvals',inf,'plotchannels',[],'stepsize',0,'downsampling',1,'loggingmode',3,'channels',1),'operator','NOT','output',struct('class','default','type','Bool8','description','','address','','unit','','name','$S_$B'),'date',731430.46749816)  Operator=NOT  Inputs=1
  Logical Operator3 : Logic  Tag=struct('inputs','2','comment',struct('text','','placement',1),'logdata',struct('maxnumvals',inf,'plotchannels',[],'stepsize',0,'downsampling',1,'loggingmode',3,'channels',1),'operator','OR','output',struct('class','default','type','Bool8','description','','address','','unit','','name','$S_$B'),'date',731430.467498704)  Operator=OR
  Switch : Switch  Criteria=u2 ~= 0
  Switch1 : Switch  Criteria=u2 ~= 0
  Terminator : Terminator
  UnitDelay : UnitDelay  Tag=struct('comment',struct('text','','placement',1),'logdata',struct('maxnumvals',inf,'plotchannels',[],'stepsize',0,'downsampling',1,'loggingmode',3,'channels',1),'output',struct('width',1,'name','$S_$B','unit','','type','Int32Bin15','offset',0,'max',32767,'min',-32768,'freeze',1,'lsb',2^-16,'arb',0,'class','default','address','','description','','autoscalingmode',1,'lowerheadroom',1,'upperheadroom',1,'headroomunit','bit','checkmin',0,'checkmax',0,'show',0,'initial','0'),'state',0,'dt','-1','date',731401.644401968)  SampleTime=-1
  fault_filter_reset : hcu_lib/fault_filter_reset
  fault_flg : Outport
  valid_signal : Outport  Port=2
  wires:
  [ifault_flg] -> fault_filter_reset/1  "ifault_flg"
  fault_filter_reset/2 -> Terminator/1  "ff_count"
  fault_filter_reset/1 -> fault_flg/1, Switch/2  "fault_flg"
  Switch/1 -> valid_signal/1, UnitDelay/1  "valid_signal"
  def_value/1 -> Switch/1  "def_value"
  Logical Operator1/1 -> Logical Operator3/1
  new_signal_valid_flg/1 -> Logical Operator1/1  "new_signal_valid_flg"
  invalid_override/1 -> Logical Operator3/2
  sat/1 -> fault_filter_reset/2  "sat"
  inc/1 -> fault_filter_reset/3  "inc"
  dec/1 -> fault_filter_reset/4  "dec"
  UnitDelay/1 -> Switch1/1  "old_signal"
  Switch1/1 -> Switch/3
  new_signal/1 -> Switch1/3  "new_signal"
  Logical Operator/1 -> [ifault_flg]  "ifault_flg"
  [ifault_flg] -> Switch1/2
  valid_override/1 -> Logical Operator2/1
  Logical Operator3/1 -> Logical Operator/1
  Logical Operator2/1 -> Logical Operator/2

== system hcu_lib/signal validity checking ==
  Signal_Raw : Inport
  Signal_Raw_valid_flg : Inport  Port=2
  invalid_override : Inport  Port=3
  valid_override : Inport  Port=4
  def_value : Inport  Port=5
  Active_fault_flg : Inport  Port=6
  Logical Operator : Logic  Tag=struct('inputs','2','comment',struct('text','','placement',1),'logdata',struct('maxnumvals',inf,'plotchannels',[],'stepsize',0,'downsampling',1,'loggingmode',3,'channels',1),'operator','OR','output',struct('class','default','type','Bool8','description','','address','','unit','','name','$S_$B'),'date',731430.467498704)
  Logical Operator1 : Logic  Tag=struct('inputs','1','comment',struct('text','','placement',1),'logdata',struct('maxnumvals',inf,'plotchannels',[],'stepsize',0,'downsampling',1,'loggingmode',3,'channels',1),'operator','NOT','output',struct('class','default','type','Bool8','description','','address','','unit','','name','$S_$B'),'date',731430.46749816)  Operator=NOT  Inputs=1
  Logical Operator2 : Logic  Tag=struct('inputs','1','comment',struct('text','','placement',1),'logdata',struct('maxnumvals',inf,'plotchannels',[],'stepsize',0,'downsampling',1,'loggingmode',3,'channels',1),'operator','NOT','output',struct('class','default','type','Bool8','description','','address','','unit','','name','$S_$B'),'date',731430.46749816)  Operator=NOT  Inputs=1
  Logical Operator3 : Logic  Tag=struct('inputs','2','comment',struct('text','','placement',1),'logdata',struct('maxnumvals',inf,'plotchannels',[],'stepsize',0,'downsampling',1,'loggingmode',3,'channels',1),'operator','OR','output',struct('class','default','type','Bool8','description','','address','','unit','','name','$S_$B'),'date',731430.467498704)  Operator=OR
  Switch : Switch  Criteria=u2 ~= 0
  Switch1 : Switch  Criteria=u2 ~= 0
  UnitDelay : UnitDelay  Tag=struct('comment',struct('text','','placement',1),'logdata',struct('maxnumvals',inf,'plotchannels',[],'stepsize',0,'downsampling',1,'loggingmode',3,'channels',1),'output',struct('width',1,'name','$S_$B','unit','','type','Int32Bin15','offset',0,'max',32767,'min',-32768,'freeze',1,'lsb',2^-16,'arb',0,'class','default','address','','description','','autoscalingmode',1,'lowerheadroom',1,'upperheadroom',1,'headroomunit','bit','checkmin',0,'checkmax',0,'show',0,'initial','0'),'state',0,'dt','-1','date',731401.644401968)  SampleTime=-1
  Short_Fault_flag : Outport
  Signal_Proc : Outport  Port=2
  wires:
  Switch/1 -> Signal_Proc/1, UnitDelay/1  "Signal_Proc"
  def_value/1 -> Switch/1  "def_value"
  Logical Operator1/1 -> Logical Operator3/1
  Signal_Raw_valid_flg/1 -> Logical Operator1/1  "Signal_Raw_valid_flg"
  invalid_override/1 -> Logical Operator3/2
  Active_fault_flg/1 -> Switch/2  "Active_fault_flg"
  UnitDelay/1 -> Switch1/1  "old_signal"
  Switch1/1 -> Switch/3
  Signal_Raw/1 -> Switch1/3  "Signal_Raw"
  Logical Operator/1 -> Short_Fault_flag/1, [ifault_flg]  "ifault_flg"
  [ifault_flg] -> Switch1/2
  valid_override/1 -> Logical Operator2/1
  Logical Operator3/1 -> Logical Operator/1
  Logical Operator2/1 -> Logical Operator/2

== system hcu_lib/signal validity checking with temp value ==
  Signal_Raw : Inport
  Signal_Raw_valid_flg : Inport  Port=2
  invalid_override : Inport  Port=3
  valid_override : Inport  Port=4
  temp_value : Inport  Port=5
  def_value : Inport  Port=6
  Active_fault_flg : Inport  Port=7
  diagnosis_switch : Inport  Port=8
  Logical Operator : Logic  Tag=struct('inputs','2','comment',struct('text','','placement',1),'logdata',struct('maxnumvals',inf,'plotchannels',[],'stepsize',0,'downsampling',1,'loggingmode',3,'channels',1),'operator','OR','output',struct('class','default','type','Bool8','description','','address','','unit','','name','$S_$B'),'date',731430.467498704)
  Logical Operator1 : Logic  Tag=struct('inputs','1','comment',struct('text','','placement',1),'logdata',struct('maxnumvals',inf,'plotchannels',[],'stepsize',0,'downsampling',1,'loggingmode',3,'channels',1),'operator','NOT','output',struct('class','default','type','Bool8','description','','address','','unit','','name','$S_$B'),'date',731430.46749816)  Operator=NOT  Inputs=1
  Logical Operator2 : Logic  Tag=struct('inputs','1','comment',struct('text','','placement',1),'logdata',struct('maxnumvals',inf,'plotchannels',[],'stepsize',0,'downsampling',1,'loggingmode',3,'channels',1),'operator','NOT','output',struct('class','default','type','Bool8','description','','address','','unit','','name','$S_$B'),'date',731430.46749816)  Operator=NOT  Inputs=1
  Logical Operator3 : Logic  Tag=struct('inputs','2','comment',struct('text','','placement',1),'logdata',struct('maxnumvals',inf,'plotchannels',[],'stepsize',0,'downsampling',1,'loggingmode',3,'channels',1),'operator','OR','output',struct('class','default','type','Bool8','description','','address','','unit','','name','$S_$B'),'date',731430.467498704)  Operator=OR
  Logical Operator4 : Logic  Tag=struct('inputs','2','comment',struct('text','','placement',1),'logdata',struct('maxnumvals',inf,'plotchannels',[],'stepsize',0,'downsampling',1,'loggingmode',3,'channels',1),'operator','OR','output',struct('class','default','type','Bool8','description','','address','','unit','','name','$S_$B'),'date',731430.467498704)
  Logical Operator5 : Logic  Tag=struct('inputs','1','comment',struct('text','','placement',1),'logdata',struct('maxnumvals',inf,'plotchannels',[],'stepsize',0,'downsampling',1,'loggingmode',3,'channels',1),'operator','NOT','output',struct('class','default','type','Bool8','description','','address','','unit','','name','$S_$B'),'date',731430.46749816)  Operator=NOT  Inputs=1
  Switch : Switch  Criteria=u2 ~= 0
  Switch1 : Switch  Criteria=u2 ~= 0
  Terminator : Terminator
  Short_Fault_flag : Outport
  Signal_Proc : Outport  Port=2
  wires:
  Logical Operator5/1 -> Switch1/3
  diagnosis_switch/1 -> Logical Operator4/2
  Logical Operator4/1 -> Short_Fault_flag/1
  Logical Operator2/1 -> Logical Operator/2
  Logical Operator3/1 -> Logical Operator/1
  valid_override/1 -> Logical Operator2/1
  [ifault_flg] -> Logical Operator5/1, Switch1/2
  Logical Operator/1 -> Logical Operator4/1, [ifault_flg]  "ifault_flg"
  Signal_Raw/1 -> Terminator/1  "Signal_Raw"
  Switch1/1 -> Switch/3
  Active_fault_flg/1 -> Switch/2  "Active_fault_flg"
  invalid_override/1 -> Logical Operator3/2
  Signal_Raw_valid_flg/1 -> Logical Operator1/1  "Signal_Raw_valid_flg"
  Logical Operator1/1 -> Logical Operator3/1
  def_value/1 -> Switch/1  "def_value"
  Switch/1 -> Signal_Proc/1  "Signal_Proc"
  temp_value/1 -> Switch1/1

== system hcu_lib/trigger signal generator ==
  Time_dur [s] : Inport
  Constant3 : Constant  Value=0
  Constant4 : Constant  Value=C_TICK_TIME_S
  Relational Operator1 : RelationalOperator  OutDataTypeStr=boolean
  Sum1 : Sum  Inputs=|++  SaturateOnIntegerOverflow=on  InputSameDT=on
  Sum2 : Sum  Inputs=+-
  Switch3 : Switch  Threshold=0.5
  Unit Delay2 : UnitDelay  SampleTime=-1
  Unit Delay3 : UnitDelay  SampleTime=-1
  Trigger_signal : Outport  OutputWhenDisabled=reset  InitialOutput=[0]
  wires:
  Sum1/1 -> Switch3/3
  Constant4/1 -> Sum1/1, Sum2/2
  Relational Operator1/1 -> Trigger_signal/1, Unit Delay3/1
  Time_dur [s]/1 -> Sum2/1
  Constant3/1 -> Switch3/1
  Switch3/1 -> Unit Delay2/1, Relational Operator1/1
  Unit Delay2/1 -> Sum1/2
  Unit Delay3/1 -> Switch3/2
  Sum2/1 -> Relational Operator1/2

== system hcu_lib/xx2kxx ==
  u : Inport
  Gain : Gain  Gain=0.001
  y : Outport
  wires:
  u/1 -> Gain/1  "u"
  Gain/1 -> y/1  "y"

== system hcu_lib/COS/km2miles1 ==
  u : Inport
  Gain : Gain  Gain=RAD2DEG
  y : Outport
  wires:
  u/1 -> Gain/1  "u"
  Gain/1 -> y/1  "y"

== system hcu_lib/Derivative/DeltaInput ==
  In1 : Inport
  function : TriggerPort  TriggerType=function-call
  Subtract : Sum  Inputs=+-
  Unit Delay : UnitDelay  SampleTime=-1
  Out1 : Outport
  wires:
  In1/1 -> Unit Delay/1, Subtract/1
  Unit Delay/1 -> Subtract/2
  Subtract/1 -> Out1/1

== system hcu_lib/SIN/km2miles1 ==
  u : Inport
  Gain : Gain  Gain=RAD2DEG
  y : Outport
  wires:
  Gain/1 -> y/1  "y"
  u/1 -> Gain/1  "u"

== system hcu_lib/Signal_Conversion_Blocks/Raw32 ==
  input : Inport
  gain : Inport  Port=2
  offset : Inport  Port=3
  Add1 : Sum  Inputs=+-
  Constant : Constant  Value=EPSILON
  Data Type Conversion6 : DataTypeConversion  OutDataTypeStr=uint32
  Divide : Product  Inputs=*/
  MinMax : MinMax  Function=max  Inputs=2
  Rounding Function : Rounding  Operator=round
  raw_value : Outport
  wires:
  Data Type Conversion6/1 -> raw_value/1
  Rounding Function/1 -> Data Type Conversion6/1
  input/1 -> Add1/1
  offset/1 -> Add1/2
  Add1/1 -> Divide/1
  Divide/1 -> Rounding Function/1
  gain/1 -> MinMax/1
  MinMax/1 -> Divide/2
  Constant/1 -> MinMax/2

== system hcu_lib/Signal_Conversion_Blocks/conv_counts_to_eng_units ==
  signal : Inport
  gain : Inport  Port=2
  offset : Inport  Port=3
  Product : Product  RndMeth=Zero
  Sum : Sum
  output_signal : Outport
  wires:
  Product/1 -> Sum/1
  gain/1 -> Product/1  "gain"
  signal/1 -> Product/2  "signal"
  offset/1 -> Sum/2  "offset"
  Sum/1 -> output_signal/1  "output_signal"

== system hcu_lib/Signal_Conversion_Blocks/conv_eng_units_to_counts ==
  input : Inport
  gain : Inport  Port=2
  offset : Inport  Port=3
  Constant : Constant  Value=0  OutDataTypeStr=Inherit: Inherit via back propagation
  Sum : Sum  Inputs=+-
  divide : hcu_lib/Basic_Blocks/divide  SystemSampleTime=-1
  output_signal : Outport
  wires:
  Constant/1 -> divide/3
  offset/1 -> Sum/2  "offset"
  input/1 -> Sum/1  "input"
  gain/1 -> divide/2  "gain"
  Sum/1 -> divide/1  "out_signal"
  divide/1 -> output_signal/1  "output_signal"

== system hcu_lib/Signal_Conversion_Blocks/convert_in ==
  raw32 : Inport
  Add : Sum
  Data Type Conversion : DataTypeConversion  OutDataTypeStr=single
  Product : Product  RndMeth=Zero
  gain : Constant  Value=single(gain)  OutDataTypeStr=single
  offset : Constant  Value=single(offset)  OutDataTypeStr=single
  value : Outport
  wires:
  raw32/1 -> Data Type Conversion/1
  gain/1 -> Product/2
  Product/1 -> Add/1
  offset/1 -> Add/2
  Add/1 -> value/1
  Data Type Conversion/1 -> Product/1

== system hcu_lib/Signal_Conversion_Blocks/convert_out ==
  value : Inport
  Add : Sum  Inputs=+-
  Constant : Constant  Value=EPSILON
  Data Type Conversion : DataTypeConversion  OutDataTypeStr=uint32  RndMeth=Nearest
  Divide : Product  Inputs=*/
  MinMax : MinMax  Function=max  Inputs=2
  gain : Constant  Value=single(gain)  OutDataTypeStr=single
  offset : Constant  Value=single(offset)  OutDataTypeStr=single
  raw32 : Outport
  wires:
  value/1 -> Add/1
  offset/1 -> Add/2
  Divide/1 -> Data Type Conversion/1
  Add/1 -> Divide/1
  Data Type Conversion/1 -> raw32/1
  gain/1 -> MinMax/1
  Constant/1 -> MinMax/2
  MinMax/1 -> Divide/2

== system hcu_lib/Signal_over/NewValue ==
  In1 : Inport
  Action Port : ActionPort
  Out1 : Outport
  wires:
  In1/1 -> Out1/1

== system hcu_lib/Signal_over/OldValue ==
  In1 : Inport
  Action Port : ActionPort
  Out1 : Outport
  wires:
  In1/1 -> Out1/1

== system hcu_lib/TAN/COS ==
  u_rad : Inport
  COS_Function : Lookup_n-D  NumberOfTableDimensions=1  BreakpointsForDimension1="[0\t5\t10\t15\t30\t45\t60\t75\t80\t85\t90\t95\t100\t105\t120\t135\t150\t165\t170\t175\t180\t185\t190\t195\t210\t225\t240\t255\t260\t265\t270\t275\t280\t285\t300\t315\t330\t345\t350\t355\t360]"  Table="[1\t0.996194698\t0.984807753\t0.965925826\t0.866025404\t0.707106781\t0.5\t0.258819045\t0.173648178\t0.087155743\t0\t-0.087155743\t-0.173648178\t-0.258819045\t-0.5\t-0.707106781\t-0.866025404\t-0.965925826\t-0.984807753\t-0.996194698\t-1\t-0.996194698\t-0.984807753\t-0.965925826\t-0.866025404\t-0.707106781\t-0.5\t-0.258819045\t-0.173648178\t-0.087155743\t0\t0.087155743\t0.173648178\t0.258819045\t0.5\t0.707106781\t0.866025404\t0.965925826\t0.984807753\t0.996194698\t1]"  ExtrapMethod=Clip  UseLastTableValue=on  InternalRulePriority=Speed  RndMeth=Simplest  InputSameDT=on
  Constant : Constant  Value=single(2*pi)
  Gain : Gain  Gain=2*pi
  Product : Product  Inputs=*/
  Rounding Function : Rounding
  Saturation : Saturate  UpperLimit=360  LowerLimit=0
  Subtract : Sum  Inputs=+-
  km2miles1 : Subsystem  mask(Conversion){}
      mask help: Convert rads to degs.
      mask Display: disp('rad \rightarrow deg', 'texmode', 'on')
  y : Outport
  wires:
  Subtract/1 -> km2miles1/1(u)
  Gain/1 -> Subtract/2
  Rounding Function/1 -> Gain/1
  Product/1 -> Rounding Function/1
  Constant/1 -> Product/2
  u_rad/1 -> Subtract/1, Product/1
  km2miles1/1(y) -> Saturation/1
  Saturation/1 -> COS_Function/1
  COS_Function/1 -> y/1

== system hcu_lib/TAN/SIN ==
  u_rad : Inport
  Constant : Constant  Value=single(2*pi)
  Gain : Gain  Gain=2*pi
  Product : Product  Inputs=*/
  Rounding Function : Rounding
  SIN_Function : Lookup_n-D  NumberOfTableDimensions=1  BreakpointsForDimension1="[0\t5\t10\t15\t30\t45\t60\t75\t80\t85\t90\t95\t100\t105\t120\t135\t150\t165\t170\t175\t180\t185\t190\t195\t210\t225\t240\t255\t260\t265\t270\t275\t280\t285\t300\t315\t330\t345\t350\t355\t360]"  Table="[0\t0.087155743\t0.173648178\t0.258819045\t0.5\t0.707106781\t0.866025404\t0.965925826\t0.984807753\t0.996194698\t1\t0.996194698\t0.984807753\t0.965925826\t0.866025404\t0.707106781\t0.5\t0.258819045\t0.173648178\t0.087155743\t0\t-0.087155743\t-0.173648178\t-0.258819045\t-0.5\t-0.707106781\t-0.866025404\t-0.965925826\t-0.984807753\t-0.996194698\t-1\t-0.996194698\t-0.984807753\t-0.965925826\t-0.866025404\t-0.707106781\t-0.5\t-0.258819045\t-0.173648178\t-0.087155743\t0]"  ExtrapMethod=Clip  UseLastTableValue=on  InternalRulePriority=Speed  RndMeth=Simplest  InputSameDT=on
  Saturation : Saturate  UpperLimit=360  LowerLimit=0
  Subtract : Sum  Inputs=+-
  km2miles1 : Subsystem  mask(Conversion){}
      mask help: Convert rads to degs.
      mask Display: disp('rad \rightarrow deg', 'texmode', 'on')
  y : Outport
  wires:
  SIN_Function/1 -> y/1
  Saturation/1 -> SIN_Function/1
  km2miles1/1(y) -> Saturation/1
  u_rad/1 -> Product/1, Subtract/1
  Constant/1 -> Product/2
  Product/1 -> Rounding Function/1
  Rounding Function/1 -> Gain/1
  Gain/1 -> Subtract/2
  Subtract/1 -> km2miles1/1(u)

== system hcu_lib/TAN/COS/km2miles1 ==
  u : Inport
  Gain : Gain  Gain=RAD2DEG
  y : Outport
  wires:
  u/1 -> Gain/1  "u"
  Gain/1 -> y/1  "y"

== system hcu_lib/TAN/SIN/km2miles1 ==
  u : Inport
  Gain : Gain  Gain=RAD2DEG
  y : Outport
  wires:
  Gain/1 -> y/1  "y"
  u/1 -> Gain/1  "u"

== stateflow chart latching fault filter reinit/lff_ctl ==
  (default) -> (junction 13)
  (junction 13) -> (junction 18) [order 1] : [reinit]
      | {fault_flg = FALSE;
      |  count = 0;}
  (junction 13) -> (junction 14) [order 2]
  (junction 14) -> (junction 15) [order 1] : [i_fault]
      | {count+=inc;}
  (junction 14) -> (junction 15) [order 2] : {count-=dec;}
  (junction 15) -> (junction 16)
  (junction 16) -> (junction 17) [order 1] : [count >= sat]
      | {count = sat;
      | fault_flg = TRUE;}
  (junction 16) -> (junction 17) [order 2] : [count <= 0]
      | {count = 0;}
  (junction 16) -> (junction 17) [order 3]
  (junction 17) -> (junction 18)
  (junction 18) -> (junction 19) : {ff_count = count;}
  data: sat input uint8; inc input uint8; dec input uint8; i_fault input boolean; fault_flg output boolean =0; ff_count output uint8; count local int16 =0; TRUE parameter boolean; FALSE parameter boolean; reinit input boolean

== stateflow chart Function Call Generator ==
  (default) -> (junction 37)
  (junction 37) -> (junction 38) [order 1] : [SampleTime_S<=C_TICK_TIME_S]
  (junction 37) -> (junction 39) [order 2] : {Timer=Timer+C_TICK_TIME_S;}
  (junction 38) -> (junction 41) : {FunCall;}
  (junction 39) -> (junction 40) [order 1] : [Timer>=SampleTime_S-0.0001]
  (junction 39) -> (junction 43) [order 2]
  (junction 40) -> (junction 42) : {FunCall;}
  (junction 41) -> (junction 45) : {Timer=0;}
  (junction 42) -> (junction 44) : {Timer=0;}
  (junction 44) -> (junction 43)
  (junction 45) -> (junction 44)
  data: SampleTime_S input double; C_TICK_TIME_S parameter double; Timer local single
  events: FunCall output FUNCTION_CALL_EVENT
